simulink model "SoRo_Compliant_Demo_0906"  (R2023b)
settings: Solver=FixedStepAuto  StartTime=0.0  StopTime=inf  FixedStep=0.01  RelTol=1e-3
undefined symbols (not defined in the file): Down, Pull
libraries: simulink x50, speedgoatlib_IO691 x20, canmsglib x19, slpidlib x12, dspfdesign x6
(part 1 of 3)
settings Model: Creator=86188  LastModifiedBy=86188
settings SolverCC: ConcurrentTasks=on  PositivePriorityOrder=on
settings OptimizationCC: BlockReduction=off  OptimizeBlockIOStorage=off  BufferReuse=off
settings DebuggingCC: AlgebraicLoopMsg=none  TasksWithSamePriorityMsg=none
settings HardwareCC: ProdBitPerLong=64  ProdLongLongMode=on  ProdHWDeviceType=Intel->x86-64 (Linux 64)
settings RTWCC: Description=Simulink Real-Time  SystemTargetFile=slrealtime.tlc  TemplateMakefile=slrealtime_default_tmf  Toolchain=Simulink Real-Time Toolchain  BuildConfiguration=Faster Runs  CodeExecutionProfiling=on  TargetLang=C++

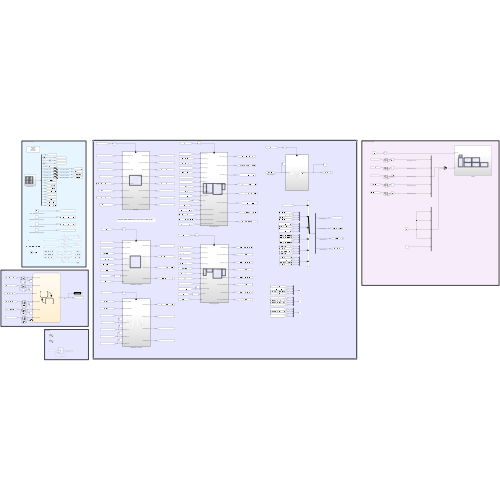
[thumbnail: Simulink's stored preview of the top-level diagram]
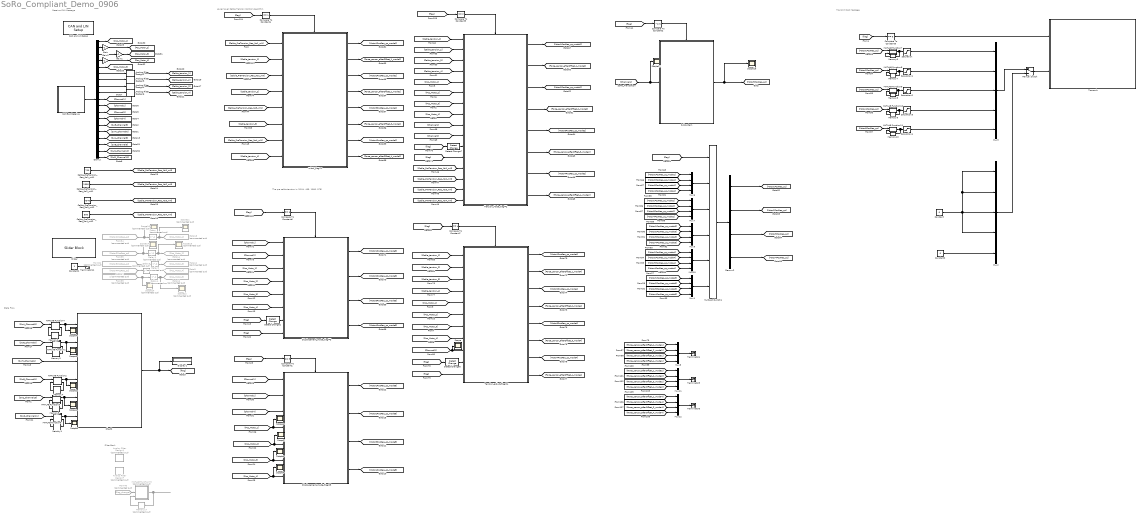
== system SoRo_Compliant_Demo_0906 ==
  note: Filter Bank
  note: Stata Flow
  note: Transmit CAN Message
  note: Receive CAN Message
  note: Lower level Cable Tension Control Algorithm
  note: The pre cable tension is (1104, 455, 1080, 978)
  Analog Filter Design1 : dspfdesign/Analog Filter Design  Commented=on  method=Chebyshev I  filttype=Lowpass  N=3  Wlo=1.5  Whi=80  Rp=2  Rs=40
  Analog Filter Design{2..4,6} (4 alike) : dspfdesign/Analog Filter Design  method=Butterworth  filttype=Lowpass  N=2  Wlo=1  Whi=80  Rp=2  Rs=40
  Analog Filter Design5 : dspfdesign/Analog Filter Design  Commented=on  method=Butterworth  filttype=Lowpass  N=3  Wlo=20  Whi=80  Rp=2  Rs=40
  CAN Bus Receive : Subsystem
  "CAN and LIN Setup " : speedgoatlib_IO691/CAN and LIN Setup   moduleInitValues="[691    1    1   -1   -1]"  id=1  moduleType=IO691  pciSlot=-1  canChn1=CAN (HS)  canChn2=CAN (HS)  canChn3=Disabled  canChn4=Disabled  linChn1=Disabled  linChn2=Disabled  canInitStructArray=[]  canTermStructArray=[]  gpioChnx=Disabled  canChn1InitValues="[2   2   8   1  16   3  19   2   2   5   2   0]"  arbBdrChn1=500 kBaud  clockDividerChn1=Enable  arbManBdrChn1=[8,1,16,3]  fdBdrChn1=5.0 MBaud  fdManBdrChn1=[2,2,5,2]  termResistor1=off  canChn2InitValues="[2   2   8   1  16   3  19   2   2   5   2   0]"  arbBdrChn2=500 kBaud  clockDividerChn2=Enable  arbManBdrChn2=[8,1,16,3]  fdBdrChn2=5.0 MBaud  fdManBdrChn2=[2,2,5,2]  termResistor2=off  canChn3InitValues="[1   0   2   8  31   8  19   2   2   5   2   0]"  arbBdrChn3=1.0 MBaud  clockDividerChn3=Enable  arbManBdrChn3=[2,8,31,8]  fdBdrChn3=5.0 MBaud  fdManBdrChn3=[2,2,5,2]  termResistor3=off  canChn4InitValues="[1   0   2   8  31   8  19   2   2   5   2   0]"  arbBdrChn4=1.0 MBaud  clockDividerChn4=Enable  arbManBdrChn4=[2,8,31,8]  fdBdrChn4=5.0 MBaud  fdManBdrChn4=[2,2,5,2]  termResistor4=off  linChn1InitValues="[0  9600]"  linBtrChn1=9600  linChn2InitValues="[0  9600]"  linBtrChn2=9600  doInitTermStruct="[0  5  0  0  0]"  parDoChannels=[1 2]  parDoVoltage=5  parDoInitValues=0  parDoReset=1  parNumOfDoS=0  parDiChannels=[3 4]  parDiVoltage=5  parDiPull=Pull-Down
      settings: SourceProductName=Simulink Real-Time: Speedgoat I/O Blockset
  Cable_PreTension_Req_No1_mN1 : Constant  Value=700
  Cable_PreTension_Req_No2_mN1 : Constant  Value=1300
  Cable_PreTension_Req_No3_mN2 : Constant  Value=7340
  Cable_PreTension_Req_No4_mN2 : Constant  Value=500
  Chart2 : Stateflow chart  TreatAsAtomicUnit=on
  Compare To Constant1 : simulink/Logic and Bit Operations/Compare To Constant  relop===  const=5  OutDataTypeStr=boolean
  Compare To Constant2 : simulink/Logic and Bit Operations/Compare To Constant  relop=~=  const=5  OutDataTypeStr=boolean
  Compare To Constant3 : simulink/Logic and Bit Operations/Compare To Constant  relop===  const=6  OutDataTypeStr=boolean
  Compare To Constant4 : simulink/Logic and Bit Operations/Compare To Constant  relop===  const=1  OutDataTypeStr=boolean
  Compare To Constant5 : simulink/Logic and Bit Operations/Compare To Constant  relop===  const=2  OutDataTypeStr=boolean
  Compare To Constant6 : simulink/Logic and Bit Operations/Compare To Constant  relop===  const=3  OutDataTypeStr=boolean
  Compare To Constant7 : simulink/Logic and Bit Operations/Compare To Constant  relop===  const=4  OutDataTypeStr=boolean
  Constant : Constant  Value=0
  Constant1 : Constant
  Constant2 : Constant  Value=0
  Delay{,1..4} (5 alike) : Delay  Commented=on
  Demux : Demux  Outputs=19
  Demux2 : Demux
  Detect Change1 : simulink/Logic and Bit Operations/Detect Change  vinit=0  OutDataTypeStr=boolean
  Detect Change6 : simulink/Logic and Bit Operations/Detect Change  vinit=0  OutDataTypeStr=boolean
  Detect Change7 : simulink/Logic and Bit Operations/Detect Change  vinit=0  OutDataTypeStr=boolean
  Displacement_mode_flag=3 : Subsystem
  Displacement_mode_flag=5 : Subsystem
  Display1 : Display
  From34 : From  Commented=on  GotoTag=Motor1PosReq_qc
  From35 : From  Commented=on  GotoTag=Motor2PosReq_qc
  From36 : From  Commented=on  GotoTag=Motor3PosReq_qc
  From37 : From  Commented=on  GotoTag=Motor4PosReq_qc
  From39 : From  Commented=on  GotoTag=Motor5PosReq_qc
  From40 : From  Commented=on  GotoTag=flag_change
  Gain : Gain  Gain=-1
  Gain1 : Gain  Gain=-1
  Gain2 : Gain  Gain=-1
  Goto12 : Goto  Commented=on  GotoTag=Pos_Motor_3
  Goto14 : Goto  Commented=on  GotoTag=Pos_Motor_2
  Goto16 : Goto  Commented=on  GotoTag=Pos_Motor_5
  Goto18 : Goto  Commented=on  GotoTag=Pos_Motor_1
  Goto9 : Goto  Commented=on  GotoTag=Pos_Motor_4
  Initial_flag=1 : Subsystem
  MATLAB Function1 : MATLAB Function  TreatAsAtomicUnit=on
  MATLAB Function10 : MATLAB Function  TreatAsAtomicUnit=on
  MATLAB Function11 : MATLAB Function  TreatAsAtomicUnit=on
  MATLAB Function13 : MATLAB Function  Commented=on  TreatAsAtomicUnit=on
  MATLAB Function2 : MATLAB Function  TreatAsAtomicUnit=on
  MATLAB Function3 : MATLAB Function  TreatAsAtomicUnit=on
  MATLAB Function4 : MATLAB Function  TreatAsAtomicUnit=on
  MATLAB Function6 : MATLAB Function  TreatAsAtomicUnit=on
  MATLAB Function7 : MATLAB Function  TreatAsAtomicUnit=on
  MATLAB Function8 : MATLAB Function  TreatAsAtomicUnit=on
  MATLAB Function9 : MATLAB Function  TreatAsAtomicUnit=on
  Manual Switch : ManualSwitch
  Memory{1..10} (10 alike) : Memory
  Memory17 : Memory  Commented=on
  Multiport Switch1 : MultiPortSwitch  Inputs=5  SaturateOnIntegerOverflow=off  InputSameDT=off
  Mux{1,6..12} (8 alike) : Mux
  Mux2 : Mux  Inputs=5
  Mux3 : Mux  Inputs=5
  Saturation{,1..3} (4 alike) : Saturate  UpperLimit=8000  LowerLimit=-8000
  Saturation4 : Saturate  UpperLimit=80000  LowerLimit=-80000
  Scope{,1..9,16..17} (12 alike) : Scope
  Scope{10..15} (6 alike) : Scope  Commented=on
  Slider : SliderBlock
  Subsystem : Subsystem
  Tension_Mode_flag=2 : Subsystem
  Tension_adjust_flag=4 : Subsystem
  Terminator{4..6,11} (4 alike) : Terminator
  Transmit : Subsystem
  wires:
  Mux8/1 -> Terminator4/1
  Tension_adjust_flag=4/5(Motor3PosReq_qc) -> [Motor3PosReq_qc_mode4]
  [flag] -> Detect Change6/1
  Demux/4 -> Gain2/1
  Tension_adjust_flag=4/1(Motor1PosReq_qc) -> [Motor1PosReq_qc_mode4]
  Tension_Mode_flag=2/8(Force_sensor_afterOffset_4) -> [Force_sensor_afterOffset_4_mode2]
  Multiport Switch1/1 -> Demux2/1
  [Motor1PosReq_qc_mode2] -> Mux7/1
  Manual Switch/1 -> Transmit/2(Input)
  [Motor2PosReq_qc_mode3] -> Mux9/2
  Tension_Mode_flag=2/1(Motor1_pos_req_qc) -> [Motor1PosReq_qc_mode2]
  [flag] -> Compare To Constant5/1
  [Motor1PosReq_qc_mode4] -> Mux10/1
  Tension_adjust_flag=4/4(Force_sensor_afterOffset_2) -> [Force_sensor_afterOffset_2_mode4]
  [Motor3PosReq_qc_mode2] -> Mux7/3
  Detect Change6/1 -> Tension_adjust_flag=4/10(flag_change)
  [Cable_tension_4] -> Tension_adjust_flag=4/4(Force_sensor_4_g)
  Tension_adjust_flag=4/3(Motor2_pos_req_qc) -> [Motor2PosReq_qc_mode4]
  [Motor2PosReq_qc_mode1] -> Mux6/2
  [Motor4PosReq_qc_mode1] -> Mux6/4
  Initial_flag=1/3(Motor2_pos_req_qc) -> [Motor2PosReq_qc_mode1]
  Mux9/1 -> Multiport Switch1/4
  Initial_flag=1/6(Force_sensor_afterOffset_3) -> [Force_sensor_afterOffset_3_mode1]
  Tension_adjust_flag=4/8(Force_sensor_afterOffset_4) -> [Force_sensor_afterOffset_4_mode4]
  [Force_sensor_afterOffset_1_mode4] -> Mux12/1
  [Force_sensor_afterOffset_1_mode1] -> Mux8/1
  [Channel3] -> Tension_adjust_flag=4/9(SoRo_Stifness_Adjust), Scope/1
  [Cable_PreTension_Req_No2_mN] -> Initial_flag=1/3(CableTension_Req_No2_mN)
  [Force_sensor_afterOffset_4_mode2] -> Mux11/4
  Initial_flag=1/5(Motor3PosReq_qc) -> [Motor3PosReq_qc_mode1]
  [Motor4PosReq_qc_mode3] -> Mux9/4
  [flag] -> Detect Change7/1
  Tension_Mode_flag=2/5(Motor3_pos_req_qc) -> [Motor3PosReq_qc_mode2]
  Compare To Constant5/1 -> Tension_Mode_flag=2/Enable
  [Force_sensor_afterOffset_2_mode2] -> Mux11/2
  [Force_sensor_afterOffset_3_mode1] -> Mux8/3
  [Motor1PosReq_qc_mode3] -> Mux9/1
  [Motor3PosReq_qc_mode3] -> Mux9/3
  [Motor2PosReq_qc_mode4] -> Mux10/2
  Tension_adjust_flag=4/7(Motor4PosReq_qc) -> [Motor4PosReq_qc_mode4]
  Tension_adjust_flag=4/6(Force_sensor_afterOffset_3) -> [Force_sensor_afterOffset_3_mode4]
  [Force_sensor_afterOffset_3_mode4] -> Mux12/3
  [flag] -> Compare To Constant4/1
  [Cable_tension_3] -> Tension_adjust_flag=4/3(Force_sensor_3_g)
  [Force_sensor_afterOffset_1_mode2] -> Mux11/1
  Mux12/1 -> Terminator6/1
  [Force_sensor_afterOffset_2_mode4] -> Mux12/2
  [Force_sensor_afterOffset_4_mode1] -> Mux8/4
  [Force_sensor_afterOffset_4_mode4] -> Mux12/4
  Displacement_mode_flag=3/3(Motor3PosReq_qc) -> [Motor3PosReq_qc_mode3]
  [Motor3PosReq_qc_mode4] -> Mux10/3
  Compare To Constant7/1 -> Tension_adjust_flag=4/Enable
  [flag] -> Tension_adjust_flag=4/11(flag)
  Mux11/1 -> Terminator5/1
  Detect Change7/1 -> Tension_Mode_flag=2/11(flag_change)
  [Cable_tension_1] -> Tension_adjust_flag=4/1(Force_sensor_1_g)
  Mux10/1 -> Multiport Switch1/5
  Displacement_mode_flag=3/2(Motor2_pos_req_qc) -> [Motor2PosReq_qc_mode3]
  Displacement_mode_flag=3/4(Motor4PosReq_qc) -> [Motor4PosReq_qc_mode3]
  [Motor3PosReq_qc] -> MATLAB Function9/1(u)
  Demux/3 -> Gain1/1
  Initial_flag=1/8(Force_sensor_afterOffset_4) -> [Force_sensor_afterOffset_4_mode1]
  [Cable_tension_2] -> Tension_adjust_flag=4/2(Force_sensor_2_g)
  [Channel2] -> Tension_Mode_flag=2/10(SoRo_Tip_Up/Down)
  Demux/7 -> Analog Filter Design3/1  "force_sensor_2_org"
  [flag] -> Compare To Constant3/1
  [Motor1PosReq_qc_mode1] -> Mux6/1
  [Cable_tension_3] -> Tension_Mode_flag=2/3(Force_sensor_3_g)
  [Channel2] -> Displacement_mode_flag=3/2(SoRo_Tip_Up/Down)
  Tension_Mode_flag=2/4(Force_sensor_afterOffset_2) -> [Force_sensor_afterOffset_2_mode2]
  Mux7/1 -> Multiport Switch1/3
  Tension_Mode_flag=2/2(Force_sensor_afterOffset_1) -> [Force_sensor_afterOffset_1_mode2]
  Tension_Mode_flag=2/3(Motor2_pos_req_qc) -> [Motor2PosReq_qc_mode2]
  [Motor4PosReq_qc_mode4] -> Mux10/4
  Displacement_mode_flag=3/1(Motor1PosReq_qc) -> [Motor1PosReq_qc_mode3]
  Initial_flag=1/7(Motor4PosReq_qc) -> [Motor4PosReq_qc_mode1]
  Tension_Mode_flag=2/7(Motor4_pos_req_qc) -> [Motor4PosReq_qc_mode2]
  [Force_sensor_afterOffset_2_mode1] -> Mux8/2
  [flag] -> Tension_Mode_flag=2/12(flag)
  [Force_sensor_afterOffset_3_mode2] -> Mux11/3
  [Cable_tension_2] -> Tension_Mode_flag=2/2(Force_sensor_2_g)
  [Cable_tension_4] -> Initial_flag=1/8(Force_sensor_4_g)
  [Channel1] -> Tension_Mode_flag=2/9(SoRo_Tip_Left/Right)
  Tension_adjust_flag=4/2(Force_sensor_afterOffset_1) -> [Force_sensor_afterOffset_1_mode4]
  Compare To Constant4/1 -> Initial_flag=1/Enable
  Tension_Mode_flag=2/6(Force_sensor_afterOffset_3) -> [Force_sensor_afterOffset_3_mode2]
  [flag] -> Compare To Constant6/1
  Mux6/1 -> Multiport Switch1/2
  [flag] -> Compare To Constant7/1
  [Cable_tension_3] -> Initial_flag=1/6(Force_sensor_3_g)
  [Motor3PosReq_qc_mode1] -> Mux6/3
  Demux/17 -> [SwB_Channel9]
  Mux2/1 -> Manual Switch/2
  Demux/1 -> [Pos_Motor_1]
  Demux/11 -> [Channel2]
  [Cable_tension_1] -> Tension_Mode_flag=2/1(Force_sensor_1_g)
  [Motor4PosReq_qc_mode2] -> Mux7/4
  [Cable_tension_4] -> Tension_Mode_flag=2/4(Force_sensor_4_g)
  [Cable_PreTension_Req_No3_mN] -> Initial_flag=1/5(CableTension_Req_No3_mN)
  Demux/16 -> [SwA_Channel8]
  [Motor2PosReq_qc_mode2] -> Mux7/2
  Compare To Constant6/1 -> Displacement_mode_flag=3/Enable
  [Cable_PreTension_Req_No1_mN] -> Initial_flag=1/1(CableTension_Req_No1_mN)
  Demux/9 -> Analog Filter Design6/1  "force_sensor_4_org"
  [Cable_tension_2] -> Initial_flag=1/4(Force_sensor_2_g)
  Demux/18 -> [SwC_Channel10]
  [Cable_tension_1] -> Initial_flag=1/2(Force_sensor_1_g)
  Demux/6 -> Analog Filter Design2/1  "force_sensor_1_org"
  Demux/13 -> [Channel4]
  Demux/15 -> [SwH_Channel6]
  Initial_flag=1/1(Motor1PosReq_qc) -> [Motor1PosReq_qc_mode1]
  [Channel1] -> Displacement_mode_flag=3/1(SoRo_Tip_Left/Right)
  Initial_flag=1/4(Force_sensor_afterOffset_2) -> [Force_sensor_afterOffset_2_mode1]
  Demux/8 -> Analog Filter Design4/1  "force_sensor_3_org"
  [Cable_PreTension_Req_No4_mN] -> Initial_flag=1/7(CableTension_Req_No4_mN)
  Demux/12 -> [Channel3]
  Initial_flag=1/2(Force_sensor_afterOffset_1) -> [Force_sensor_afterOffset_1_mode1]
  Demux/14 -> [SwE_Channel5]
  Demux/2 -> Gain/1
  CAN Bus Receive/1(Outport) -> Demux/1
  Demux/5 -> [Pos_Motor_5]
  Demux/10 -> [Channel1]
  [flag] -> Multiport Switch1/1
  MATLAB Function3/1(y) -> Chart2/5(Switch_C_Change), Scope1/1
  Memory5/1 -> MATLAB Function3/2(u_last)
  MATLAB Function4/1(y) -> Scope4/1, Chart2/1(Switch_A_Change)
  MATLAB Function3/2(u_out) -> Memory5/1
  MATLAB Function1/2(u_out) -> Memory3/1
  [SwC_Channel10] -> MATLAB Function3/1(u)
  MATLAB Function4/2(u_out) -> Memory2/1
  MATLAB Function2/2(u_out) -> Memory4/1
  Chart2/1(flag) -> Display1/1, [flag]  "flag"
  [SwH_Channel6] -> Chart2/3(Switch_H)
  MATLAB Function1/1(y) -> Scope3/1, Chart2/2(Switch_E_Change)
  Memory4/1 -> MATLAB Function2/2(u_last)
  [SwB_Channel9] -> MATLAB Function2/1(u)
  [SwA_Channel8] -> MATLAB Function4/1(u)
  Memory2/1 -> MATLAB Function4/2(u_last)
  Memory3/1 -> MATLAB Function1/2(u_last)
  [SwE_Channel5] -> MATLAB Function1/1(u)
  MATLAB Function2/1(y) -> Scope2/1, Chart2/4(Switch_B_Change)
  Compare To Constant3/1 -> Transmit/1(End Test)
  [Pos_Motor_2] -> Tension_Mode_flag=2/6(Pos_Motor_2_qc)
  [Pos_Motor_3] -> Tension_Mode_flag=2/7(Pos_Motor_3_qc)
  [Pos_Motor_4] -> Tension_Mode_flag=2/8(Pos_Motor_4_qc)
  [Pos_Motor_1] -> Tension_Mode_flag=2/5(Pos_Motor_1_qc)
  [Pos_Motor_3] -> Tension_adjust_flag=4/7(Pos_Motor_3_qc)
  [Pos_Motor_2] -> Tension_adjust_flag=4/6(Pos_Motor_2_qc)
  [Pos_Motor_4] -> Tension_adjust_flag=4/8(Pos_Motor_4_qc)
  [Pos_Motor_1] -> Tension_adjust_flag=4/5(Pos_Motor_1_qc)
  [Pos_Motor_2] -> Displacement_mode_flag=3/4(Pos_Motor_2_qc)
  [Pos_Motor_1] -> Displacement_mode_flag=3/3(Pos_Motor_1_qc)
  [Pos_Motor_3] -> Displacement_mode_flag=3/5(Pos_Motor_3_qc)
  [Pos_Motor_4] -> Displacement_mode_flag=3/6(Pos_Motor_4_qc)
  [flag] -> Detect Change1/1
  [flag] -> Displacement_mode_flag=3/8(flag)
  Detect Change1/1 -> Displacement_mode_flag=3/7(flag_change)
  Constant1/1 -> Terminator11/1
  MATLAB Function6/2(u_out) -> Memory1/1
  MATLAB Function6/1(y) -> Chart2/6(Switch_D_Change), Scope5/1
  [SwD_Channel11] -> MATLAB Function6/1(u)
  Memory1/1 -> MATLAB Function6/2(u_last)
  Demux/19 -> [SwD_Channel11]
  [Pos_Motor_1] -> Scope6/1, Displacement_mode_flag=5/4(Pos_Motor_1_qc)
  [Pos_Motor_4] -> Scope9/1, Displacement_mode_flag=5/7(Pos_Motor_4_qc)
  [flag] -> Compare To Constant1/1
  [Pos_Motor_3] -> Scope8/1, Displacement_mode_flag=5/6(Pos_Motor_3_qc)
  [Pos_Motor_2] -> Scope7/1, Displacement_mode_flag=5/5(Pos_Motor_2_qc)
  [Channel2] -> Displacement_mode_flag=5/2(UpMotor3_DownMotor2)
  [Channel1] -> Displacement_mode_flag=5/1(LeftMotor4_RightMotor1)
  Compare To Constant1/1 -> Displacement_mode_flag=5/Enable
  Displacement_mode_flag=5/1(Motor1PosReq_qc) -> [Motor1PosReq_qc_mode5]
  Displacement_mode_flag=5/3(Motor3PosReq_qc) -> [Motor3PosReq_qc_mode5]
  Displacement_mode_flag=5/4(Motor4PosReq_qc) -> [Motor4PosReq_qc_mode5]
  Displacement_mode_flag=5/2(Motor2_pos_req_qc) -> [Motor2PosReq_qc_mode5]
  [Channel4] -> Displacement_mode_flag=5/3(Pos_IncreaseDecrease)
  [Motor4PosReq_qc_mode5] -> Mux1/4
  [Motor3PosReq_qc_mode5] -> Mux1/3
  Mux1/1 -> Multiport Switch1/6
  [Motor2PosReq_qc_mode5] -> Mux1/2
  [Motor1PosReq_qc_mode5] -> Mux1/1
  Saturation4/1 -> Mux3/5  "Motor5PosReq_qc_final"
  Mux3/1 -> Manual Switch/1
  Saturation3/1 -> Mux3/4  "Motor4PosReq_qc_final"
  Saturation/1 -> Mux3/1  "Motor1PosReq_qc_final"
  Saturation1/1 -> Mux3/2  "Motor2PosReq_qc_final"
  Saturation2/1 -> Mux3/3  "Motor3PosReq_qc_final"
  [Motor1PosReq_qc] -> MATLAB Function7/1(u)
  MATLAB Function7/1(y) -> Memory6/1, Saturation/1
  Memory6/1 -> MATLAB Function7/2(u_last)
  MATLAB Function9/1(y) -> Memory8/1, Saturation2/1
  MATLAB Function8/1(y) -> Memory7/1, Saturation1/1
  [Motor2PosReq_qc] -> MATLAB Function8/1(u)
  Memory7/1 -> MATLAB Function8/2(u_last)
  Memory8/1 -> MATLAB Function9/2(u_last)
  MATLAB Function10/1(y) -> Memory9/1, Saturation3/1
  [Motor4PosReq_qc] -> MATLAB Function10/1(u)
  Memory9/1 -> MATLAB Function10/2(u_last)
  MATLAB Function11/1(y) -> Memory10/1, Saturation4/1
  Memory10/1 -> MATLAB Function11/2(u_last)
  From39/1 -> Delay4/1, Scope13/1
  From35/1 -> Delay1/1, Scope14/1
  From36/1 -> Delay2/1
  From37/1 -> Delay3/1
  Delay/1 -> Scope11/1, Goto18/1
  Delay1/1 -> Goto14/1, Scope15/1
  Delay2/1 -> Goto12/1
  Delay3/1 -> Goto9/1
  Delay4/1 -> Scope12/1, Goto16/1
  From40/1 -> MATLAB Function13/2(change)
  Memory17/1 -> MATLAB Function13/3(u_last)
  MATLAB Function13/1(y) -> Memory17/1  "Motor2PosReq_qc"
  Demux2/1 -> [Motor1PosReq_qc]  "Motor1PosReq_qc"
  Demux2/2 -> [Motor2PosReq_qc]  "Motor2PosReq_qc"
  Demux2/3 -> [Motor3PosReq_qc]  "Motor3PosReq_qc"
  Demux2/4 -> [Motor4PosReq_qc]  "Motor4PosReq_qc"
  From34/1 -> Scope10/1, Delay/1
  [Motor5PosReq_qc] -> MATLAB Function11/1(u)
  [Channel4] -> Scope17/1, Subsystem/1(Channel4)
  [flag] -> Compare To Constant2/1
  Compare To Constant2/1 -> Subsystem/Enable
  Subsystem/1(Motor5PosReq_qc) -> Scope16/1, [Motor5PosReq_qc]
  Analog Filter Design2/1 -> [Cable_tension_1]  "force_sensor_1_filtered"
  Analog Filter Design3/1 -> [Cable_tension_2]  "force_sensor_2_filtered"
  Analog Filter Design4/1 -> [Cable_tension_3]  "force_sensor_3_filtered"
  Analog Filter Design6/1 -> [Cable_tension_4]  "force_sensor_4_filtered"
  Constant/1 -> Mux2/4, Mux2/1, Mux2/2, Mux2/3
  Constant2/1 -> Mux2/5
  Gain/1 -> [Pos_Motor_2]
  Gain1/1 -> [Pos_Motor_3]
  Gain2/1 -> [Pos_Motor_4]
  Cable_PreTension_Req_No1_mN1/1 -> [Cable_PreTension_Req_No1_mN]
  Cable_PreTension_Req_No2_mN1/1 -> [Cable_PreTension_Req_No2_mN]
  Cable_PreTension_Req_No3_mN2/1 -> [Cable_PreTension_Req_No3_mN]
  Cable_PreTension_Req_No4_mN2/1 -> [Cable_PreTension_Req_No4_mN]
  [Cable_PreTension_Req_No1_mN] -> Tension_Mode_flag=2/13(Cable_PreTension_Req_No1_mN)
  [Cable_PreTension_Req_No2_mN] -> Tension_Mode_flag=2/14(Cable_PreTension_Req_No2_mN)
  [Cable_PreTension_Req_No3_mN] -> Tension_Mode_flag=2/15(Cable_PreTension_Req_No3_mN)
  [Cable_PreTension_Req_No4_mN] -> Tension_Mode_flag=2/16(Cable_PreTension_Req_No4_mN)

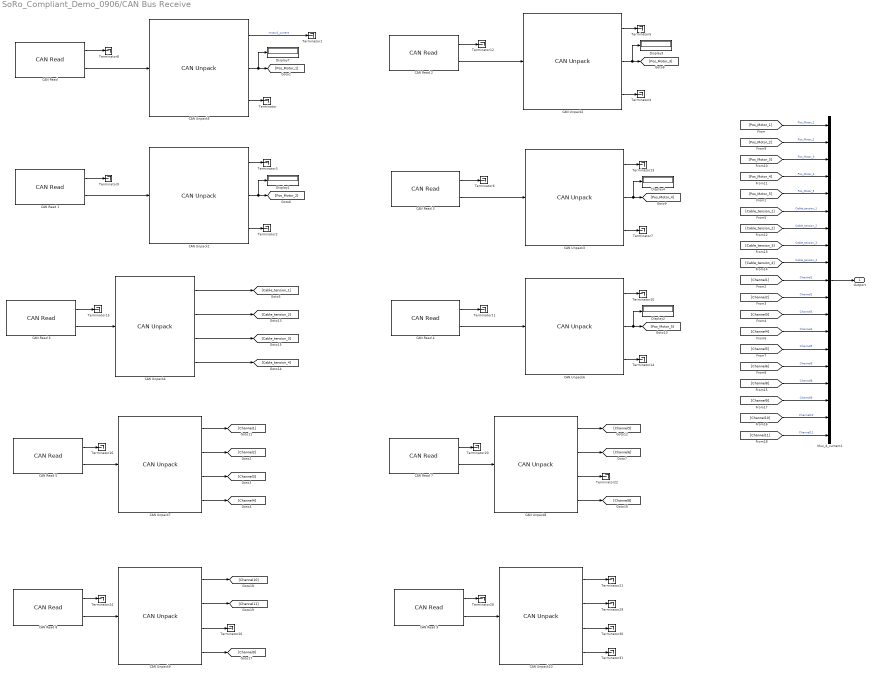
== system SoRo_Compliant_Demo_0906/CAN Bus Receive ==
  "CAN Read " : speedgoatlib_IO691/CAN Read   moduleType=IO691  id=1  channel=1  canType=CAN (HS)  messageType=CAN (HS)  useBusOut=off  HasMulRead=Specify by IDs  MsgIDlist=[27]  isEFF=off  LabelInHex=on  enableInput=off  initValues=[691 1 0.01 0 1 1 0 0 2 0 1 27]  ts=0.01
      settings: SourceProductName=Simulink Real-Time: Speedgoat I/O Blockset
  CAN Read 1 : speedgoatlib_IO691/CAN Read   moduleType=IO691  id=1  channel=1  canType=CAN (HS)  messageType=CAN (HS)  useBusOut=off  HasMulRead=Specify by IDs  MsgIDlist=[43]  isEFF=off  LabelInHex=on  enableInput=off  initValues=[691 1 0.01 0 1 1 0 0 2 0 1 43]  ts=0.01
      settings: SourceProductName=Simulink Real-Time: Speedgoat I/O Blockset
  CAN Read 2 : speedgoatlib_IO691/CAN Read   moduleType=IO691  id=1  channel=1  canType=CAN (HS)  messageType=CAN (HS)  useBusOut=off  HasMulRead=Specify by IDs  MsgIDlist=[59]  isEFF=off  LabelInHex=on  enableInput=off  initValues=[691 1 0.01 0 1 1 0 0 2 0 1 59]  ts=0.01
      settings: SourceProductName=Simulink Real-Time: Speedgoat I/O Blockset
  CAN Read 3 : speedgoatlib_IO691/CAN Read   moduleType=IO691  id=1  channel=1  canType=CAN (HS)  messageType=CAN (HS)  useBusOut=off  HasMulRead=Specify by IDs  MsgIDlist=[75]  isEFF=off  LabelInHex=on  enableInput=off  initValues=[691 1 0.01 0 1 1 0 0 2 0 1 75]  ts=0.01
      settings: SourceProductName=Simulink Real-Time: Speedgoat I/O Blockset
  CAN Read 4 : speedgoatlib_IO691/CAN Read   moduleType=IO691  id=1  channel=1  canType=CAN (HS)  messageType=CAN (HS)  useBusOut=off  HasMulRead=Specify by IDs  MsgIDlist=[91]  isEFF=off  LabelInHex=on  enableInput=off  initValues=[691 1 0.01 0 1 1 0 0 2 0 1 91]  ts=0.01
      settings: SourceProductName=Simulink Real-Time: Speedgoat I/O Blockset
  CAN Read 5 : speedgoatlib_IO691/CAN Read   moduleType=IO691  id=1  channel=1  canType=CAN (HS)  messageType=CAN (HS)  useBusOut=off  HasMulRead=Specify by IDs  MsgIDlist=[391]  isEFF=off  LabelInHex=on  enableInput=off  initValues=[691 1 0.01 0 1 1 0 0 2 0 1 391]  ts=0.01
      settings: SourceProductName=Simulink Real-Time: Speedgoat I/O Blockset
  CAN Read 6 : speedgoatlib_IO691/CAN Read   moduleType=IO691  id=1  channel=1  canType=CAN (HS)  messageType=CAN (HS)  useBusOut=off  HasMulRead=Specify by IDs  MsgIDlist=[529024]  isEFF=on  LabelInHex=on  enableInput=off  initValues=[691 1 0.01 0 1 1 0 0 2 1 1 529024]  ts=0.01
      settings: SourceProductName=Simulink Real-Time: Speedgoat I/O Blockset
  CAN Read 7 : speedgoatlib_IO691/CAN Read   moduleType=IO691  id=1  channel=1  canType=CAN (HS)  messageType=CAN (HS)  useBusOut=off  HasMulRead=Specify by IDs  MsgIDlist=[392]  isEFF=off  LabelInHex=on  enableInput=off  initValues=[691 1 0.01 0 1 1 0 0 2 0 1 392]  ts=0.01
      settings: SourceProductName=Simulink Real-Time: Speedgoat I/O Blockset
  CAN Read 8 : speedgoatlib_IO691/CAN Read   moduleType=IO691  id=1  channel=1  canType=CAN (HS)  messageType=CAN (HS)  useBusOut=off  HasMulRead=Specify by IDs  MsgIDlist=[393]  isEFF=off  LabelInHex=on  enableInput=off  initValues=[691 1 0.01 0 1 1 0 0 2 0 1 393]  ts=0.01
      settings: SourceProductName=Simulink Real-Time: Speedgoat I/O Blockset
  CAN Read 9 : speedgoatlib_IO691/CAN Read   moduleType=IO691  id=1  channel=1  canType=CAN (HS)  messageType=CAN (HS)  useBusOut=off  HasMulRead=Specify by IDs  MsgIDlist=[394]  isEFF=off  LabelInHex=on  enableInput=off  initValues=[691 1 0.01 0 1 1 0 0 2 0 1 394]  ts=0.01
      settings: SourceProductName=Simulink Real-Time: Speedgoat I/O Blockset
  CAN Unpack1 : canmsglib/CAN Unpack  CANdbFile=E:\OneDrive\OneDrive - The Chinese University of Hong Kong\文档\Research\SRIL\12nd\Experiment\Simulink\RoboModule0729.dbc  MsgList=Feedback_curvelpos_Dv2  MsgName=Feedback_curvelpos_Dv2  MsgIDType=Standard (11-bit identifier)  MsgIdentifier=43  MsgLength=8  SignalInfo={'real_current','8','16','BE','signed','Standard','0','1','0','-Inf','Inf';'real_position','56','32','BE','signed','Standard','0','1','0','-Inf','Inf';'real_velocity','24','16','BE','signed','Standard','0','1','0','-Inf','Inf'}  IDPort=off  TimestampPort=off  ErrorPort=off  RemotePort=off  LengthPort=off  StatusPort=off  ApplyMinMax=off
      settings: DataFormat=CANdb specified signals
  CAN Unpack10 : canmsglib/CAN Unpack  CANdbFile=E:\OneDrive\OneDrive - The Chinese University of Hong Kong\文档\Research\SRIL\12nd\Experiment\Simulink\RoboModule0729.dbc  MsgList=RadioLink_4  MsgName=RadioLink_4  MsgIDType=Standard (11-bit identifier)  MsgIdentifier=394  MsgLength=8  SignalInfo={'Channel13','8','16','BE','unsigned','Standard','0','1','0','-Inf','Inf';'Channel14','24','16','BE','unsigned','Standard','0','1','0','-Inf','Inf';'Channel15','40','16','BE','unsigned','Standard','0','1','0','-Inf','Inf';'Channel16','56','16','BE','unsigned','Standard','0','1','0','-Inf','Inf'}  IDPort=off  TimestampPort=off  ErrorPort=off  RemotePort=off  LengthPort=off  StatusPort=off  ApplyMinMax=off
      settings: DataFormat=CANdb specified signals
  CAN Unpack2 : canmsglib/CAN Unpack  CANdbFile=E:\OneDrive\OneDrive - The Chinese University of Hong Kong\文档\Research\SRIL\12nd\Experiment\Simulink\RoboModule0729.dbc  MsgList=Feedback_curvelpos_Dv3  MsgName=Feedback_curvelpos_Dv3  MsgIDType=Standard (11-bit identifier)  MsgIdentifier=59  MsgLength=8  SignalInfo={'real_current','8','16','BE','signed','Standard','0','1','0','-Inf','Inf';'real_position','56','32','BE','signed','Standard','0','1','0','-Inf','Inf';'real_velocity','24','16','BE','signed','Standard','0','1','0','-Inf','Inf'}  IDPort=off  TimestampPort=off  ErrorPort=off  RemotePort=off  LengthPort=off  StatusPort=off  ApplyMinMax=off
      settings: DataFormat=CANdb specified signals
  CAN Unpack3 : canmsglib/CAN Unpack  CANdbFile=E:\OneDrive\OneDrive - The Chinese University of Hong Kong\文档\Research\SRIL\12nd\Experiment\Simulink\RoboModule0729.dbc  MsgList=Feedback_curvelpos_Dr4  MsgName=Feedback_curvelpos_Dr4  MsgIDType=Standard (11-bit identifier)  MsgIdentifier=75  MsgLength=8  SignalInfo={'real_current','8','16','BE','signed','Standard','0','1','0','-Inf','Inf';'real_position','56','32','BE','signed','Standard','0','1','0','-Inf','Inf';'real_velocity','24','16','BE','signed','Standard','0','1','0','-Inf','Inf'}  IDPort=off  TimestampPort=off  ErrorPort=off  RemotePort=off  LengthPort=off  StatusPort=off  ApplyMinMax=off
      settings: DataFormat=CANdb specified signals
  CAN Unpack4 : canmsglib/CAN Unpack  CANdbFile=E:\OneDrive\OneDrive - The Chinese University of Hong Kong\文档\Research\SRIL\12nd\Experiment\Simulink\RoboModule0729.dbc  MsgList=Cable_tension  MsgName=Cable_tension  MsgIDType=Extended (29-bit identifier)  MsgIdentifier=529024  MsgLength=8  SignalInfo={'Force_sensor_1','8','16','BE','unsigned','Standard','0','1','0','-Inf','Inf';'Force_sensor_2','24','16','BE','unsigned','Standard','0','1','0','-Inf','Inf';'Force_sensor_3','40','16','BE','unsigned','Standard','0','1','0','-Inf','Inf';'Force_sensor_4','56','16','BE','unsigned','Standard','0','1','0','-Inf','Inf'}  IDPort=off  TimestampPort=off  ErrorPort=off  RemotePort=off  LengthPort=off  StatusPort=off  ApplyMinMax=off
      settings: DataFormat=CANdb specified signals
  CAN Unpack5 : canmsglib/CAN Unpack  CANdbFile=E:\OneDrive\OneDrive - The Chinese University of Hong Kong\文档\Research\SRIL\12nd\Experiment\Simulink\RoboModule0729.dbc  MsgList=Feedback_curvelpos_Dv1  MsgName=Feedback_curvelpos_Dv1  MsgIDType=Standard (11-bit identifier)  MsgIdentifier=27  MsgLength=8  SignalInfo={'real_current','8','16','BE','signed','Standard','0','1','0','-Inf','Inf';'real_position','56','32','BE','signed','Standard','0','1','0','-Inf','Inf';'real_velocity','24','16','BE','signed','Standard','0','1','0','-Inf','Inf'}  IDPort=off  TimestampPort=off  ErrorPort=off  RemotePort=off  LengthPort=off  StatusPort=off  ApplyMinMax=off
      settings: DataFormat=CANdb specified signals
  CAN Unpack6 : canmsglib/CAN Unpack  CANdbFile=E:\OneDrive\OneDrive - The Chinese University of Hong Kong\文档\Research\SRIL\12nd\Experiment\Simulink\RoboModule0729.dbc  MsgList=Feedback_curvelpos_Dr5  MsgName=Feedback_curvelpos_Dr5  MsgIDType=Standard (11-bit identifier)  MsgIdentifier=91  MsgLength=8  SignalInfo={'real_current','8','16','BE','signed','Standard','0','1','0','-Inf','Inf';'real_position','56','32','BE','signed','Standard','0','1','0','-Inf','Inf';'real_velocity','24','16','BE','signed','Standard','0','1','0','-Inf','Inf'}  IDPort=off  TimestampPort=off  ErrorPort=off  RemotePort=off  LengthPort=off  StatusPort=off  ApplyMinMax=off
      settings: DataFormat=CANdb specified signals
  CAN Unpack7 : canmsglib/CAN Unpack  CANdbFile=E:\OneDrive\OneDrive - The Chinese University of Hong Kong\文档\Research\SRIL\12nd\Experiment\Simulink\RoboModule0729.dbc  MsgList=RadioLink_1  MsgName=RadioLink_1  MsgIDType=Standard (11-bit identifier)  MsgIdentifier=391  MsgLength=8  SignalInfo={'Channel1','8','16','BE','unsigned','Standard','0','1','0','-Inf','Inf';'Channel2','24','16','BE','unsigned','Standard','0','1','0','-Inf','Inf';'Channel3','40','16','BE','unsigned','Standard','0','1','0','-Inf','Inf';'Channel4','56','16','BE','unsigned','Standard','0','1','0','-Inf','Inf'}  IDPort=off  TimestampPort=off  ErrorPort=off  RemotePort=off  LengthPort=off  StatusPort=off  ApplyMinMax=off
      settings: DataFormat=CANdb specified signals
  CAN Unpack8 : canmsglib/CAN Unpack  CANdbFile=E:\OneDrive\OneDrive - The Chinese University of Hong Kong\文档\Research\SRIL\12nd\Experiment\Simulink\RoboModule0729.dbc  MsgList=RadioLink_2  MsgName=RadioLink_2  MsgIDType=Standard (11-bit identifier)  MsgIdentifier=392  MsgLength=8  SignalInfo={'Channel5','8','16','BE','unsigned','Standard','0','1','0','-Inf','Inf';'Channel6','24','16','BE','unsigned','Standard','0','1','0','-Inf','Inf';'Channel7','40','16','BE','unsigned','Standard','0','1','0','-Inf','Inf';'Channel8','56','16','BE','unsigned','Standard','0','1','0','-Inf','Inf'}  IDPort=off  TimestampPort=off  ErrorPort=off  RemotePort=off  LengthPort=off  StatusPort=off  ApplyMinMax=off
      settings: DataFormat=CANdb specified signals
  CAN Unpack9 : canmsglib/CAN Unpack  CANdbFile=E:\Research\SRIL\12nd\Simulink\RoboModule0729.dbc  MsgList=RadioLink_3  MsgName=RadioLink_3  MsgIDType=Standard (11-bit identifier)  MsgIdentifier=393  MsgLength=8  SignalInfo={'Channel10','24','16','BE','unsigned','Standard','0','1','0','-Inf','Inf';'Channel11','40','16','BE','unsigned','Standard','0','1','0','-Inf','Inf';'Channel12','56','16','BE','unsigned','Standard','0','1','0','-Inf','Inf';'Channel9','8','16','BE','unsigned','Standard','0','1','0','-Inf','Inf'}  IDPort=off  TimestampPort=off  ErrorPort=off  RemotePort=off  LengthPort=off  StatusPort=off  ApplyMinMax=off
      settings: DataFormat=CANdb specified signals
  Display{1..4,7} (5 alike) : Display
      settings: Format=hex (Stored Integer)
  Mux_4_current1 : Mux  Inputs=19
  Terminator{,1..16,20..22,24,26,28..31} (26 alike) : Terminator
  Outport : Outport
  wires:
  CAN Unpack5/3 -> Terminator/1
  CAN Unpack4/1 -> [Cable_tension_1]
  CAN Unpack5/1 -> Terminator1/1  "motor1_current"
  "CAN Read "/2 -> CAN Unpack5/1
  CAN Unpack4/2 -> [Cable_tension_2]
  CAN Unpack5/2 -> Display7/1, [Pos_Motor_1]
  "CAN Read "/1 -> Terminator8/1
  CAN Read 1/2 -> CAN Unpack1/1
  CAN Read 1/1 -> Terminator9/1
  CAN Unpack1/2 -> Display1/1, [Pos_Motor_2]
  CAN Unpack1/3 -> Terminator2/1
  CAN Unpack1/1 -> Terminator3/1
  CAN Read 2/2 -> CAN Unpack2/1
  CAN Read 2/1 -> Terminator12/1
  CAN Unpack2/3 -> Terminator4/1
  CAN Unpack2/2 -> Display3/1, [Pos_Motor_3]
  CAN Unpack2/1 -> Terminator5/1
  CAN Read 3/2 -> CAN Unpack3/1
  CAN Unpack3/3 -> Terminator7/1
  CAN Read 3/1 -> Terminator6/1
  CAN Unpack3/1 -> Terminator13/1
  CAN Unpack3/2 -> Display4/1, [Pos_Motor_4]
  CAN Unpack6/2 -> Display2/1, [Pos_Motor_5]
  CAN Read 4/2 -> CAN Unpack6/1
  CAN Unpack6/1 -> Terminator10/1
  CAN Read 4/1 -> Terminator11/1
  CAN Unpack6/3 -> Terminator14/1
  CAN Read 6/1 -> Terminator15/1
  CAN Read 6/2 -> CAN Unpack4/1
  CAN Read 5/1 -> Terminator16/1
  CAN Read 5/2 -> CAN Unpack7/1
  CAN Unpack7/1 -> [Channel1]
  CAN Unpack7/2 -> [Channel2]
  CAN Unpack7/3 -> [Channel3]
  CAN Unpack7/4 -> [Channel4]
  CAN Unpack8/4 -> [Channel8]
  CAN Read 7/1 -> Terminator20/1
  CAN Unpack8/1 -> [Channel5]
  CAN Unpack8/2 -> [Channel6]
  CAN Read 7/2 -> CAN Unpack8/1
  CAN Unpack8/3 -> Terminator22/1
  CAN Unpack9/3 -> Terminator26/1
  CAN Unpack9/1 -> [Channel10]
  CAN Read 8/2 -> CAN Unpack9/1
  CAN Read 8/1 -> Terminator24/1
  CAN Unpack9/2 -> [Channel11]
  CAN Unpack9/4 -> [Channel9]
  CAN Unpack10/2 -> Terminator29/1
  CAN Read 9/1 -> Terminator28/1
  CAN Unpack10/4 -> Terminator31/1
  CAN Read 9/2 -> CAN Unpack10/1
  CAN Unpack10/3 -> Terminator30/1
  CAN Unpack10/1 -> Terminator21/1
  [Channel1] -> Mux_4_current1/10  "Channel1"
  [Channel2] -> Mux_4_current1/11  "Channel2"
  [Channel4] -> Mux_4_current1/13  "Channel4"
  [Channel3] -> Mux_4_current1/12  "Channel3"
  [Channel5] -> Mux_4_current1/14  "Channel5"
  [Channel6] -> Mux_4_current1/15  "Channel6"
  CAN Unpack4/4 -> [Cable_tension_4]
  CAN Unpack4/3 -> [Cable_tension_3]
  [Pos_Motor_1] -> Mux_4_current1/1  "Pos_Motor_1"
  Mux_4_current1/1 -> Outport/1
  [Pos_Motor_2] -> Mux_4_current1/2  "Pos_Motor_2"
  [Pos_Motor_3] -> Mux_4_current1/3  "Pos_Motor_3"
  [Pos_Motor_4] -> Mux_4_current1/4  "Pos_Motor_4"
  [Pos_Motor_5] -> Mux_4_current1/5  "Pos_Motor_5"
  [Cable_tension_1] -> Mux_4_current1/6  "Cable_tension_1"
  [Cable_tension_2] -> Mux_4_current1/7  "Cable_tension_2"
  [Cable_tension_3] -> Mux_4_current1/8  "Cable_tension_3"
  [Cable_tension_4] -> Mux_4_current1/9  "Cable_tension_4"
  [Channel8] -> Mux_4_current1/16  "Channel8"
  [Channel10] -> Mux_4_current1/18  "Channel10"
  [Channel9] -> Mux_4_current1/17  "Channel9"
  [Channel11] -> Mux_4_current1/19  "Channel11"

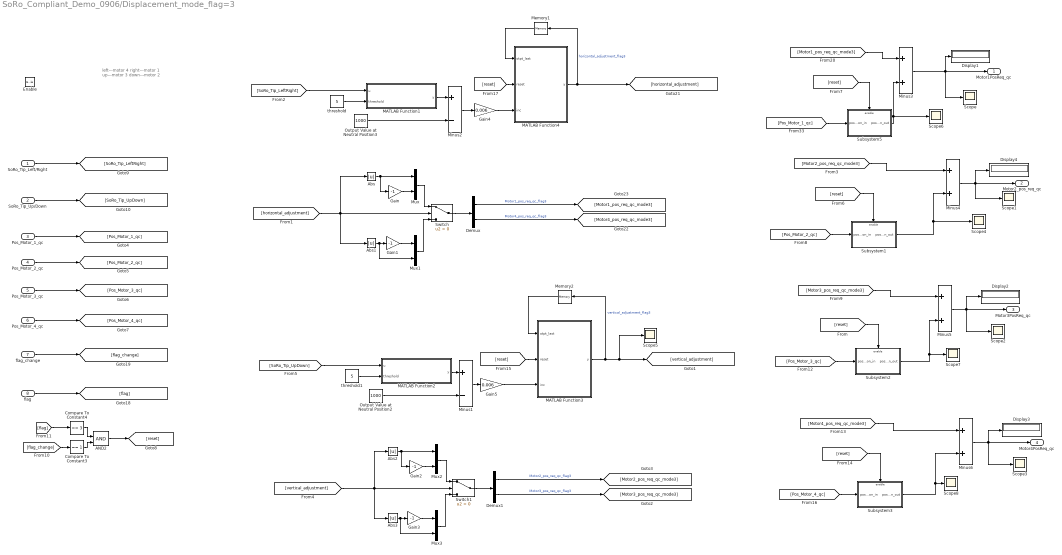
== system SoRo_Compliant_Demo_0906/Displacement_mode_flag=3 ==
  note: left---motor 4
      | right---motor 1
      | up---motor 3
      | down---motor 2
  SoRo_Tip_Left/Right : Inport
  SoRo_Tip_Up/Down : Inport  Port=2
  Pos_Motor_1_qc : Inport  Port=3
  Pos_Motor_2_qc : Inport  Port=4
  Pos_Motor_3_qc : Inport  Port=5
  Pos_Motor_4_qc : Inport  Port=6
  flag_change : Inport  Port=7
  flag : Inport  Port=8
  Enable : EnablePort  StatesWhenEnabling=reset
  AND2 : Logic  IconShape=distinctive  AllPortsSameDT=off  OutDataTypeStr=boolean
  Abs{,1..3} (4 alike) : Abs  SaturateOnIntegerOverflow=off
  Compare To Constant3 : simulink/Logic and Bit Operations/Compare To Constant  relop===  const=1  OutDataTypeStr=boolean
  Compare To Constant4 : simulink/Logic and Bit Operations/Compare To Constant  relop===  const=3  OutDataTypeStr=boolean
  Demux : Demux  Outputs=2
  Demux1 : Demux  Outputs=2
  Display{1..4} (4 alike) : Display
  Gain{,1..3} (4 alike) : Gain  Gain=-1
  Gain4 : Gain  Gain=0.006
  Gain5 : Gain  Gain=0.006
  MATLAB Function1 : MATLAB Function  TreatAsAtomicUnit=on
  MATLAB Function2 : MATLAB Function  TreatAsAtomicUnit=on
  MATLAB Function3 : MATLAB Function  TreatAsAtomicUnit=on
  MATLAB Function4 : MATLAB Function  TreatAsAtomicUnit=on
  Memory1 : Memory
  Memory2 : Memory
  Minus1 : Sum  Inputs=+-
  Minus2 : Sum  Inputs=+-
  Minus{3..6} (4 alike) : Sum
  Mux{,1..3} (4 alike) : Mux  Inputs=2
  Output Value at Neutral Position2 : Constant  Value=1000
  Output Value at Neutral Position3 : Constant  Value=1000
  Scope{,1..8} (9 alike) : Scope
  Subsystem1 : Subsystem
  Subsystem2 : Subsystem
  Subsystem3 : Subsystem
  Subsystem5 : Subsystem
  Switch : Switch  Criteria=u2 > Threshold  SaturateOnIntegerOverflow=off  InputSameDT=off
  Switch1 : Switch  Criteria=u2 > Threshold  SaturateOnIntegerOverflow=off  InputSameDT=off
  threshold : Constant  Value=5
  threshold1 : Constant  Value=5
  Motor1PosReq_qc : Outport
  Motor2_pos_req_qc : Outport  Port=2
  Motor3PosReq_qc : Outport  Port=3
  Motor4PosReq_qc : Outport  Port=4
  wires:
  SoRo_Tip_Left/Right/1 -> [SoRo_Tip_LeftRight]
  SoRo_Tip_Up/Down/1 -> [SoRo_Tip_UpDown]
  Minus2/1 -> Gain4/1
  Demux/1 -> [Motor1_pos_req_qc_mode3]  "Motor1_pos_req_qc_flag3"
  Demux/2 -> [Motor4_pos_req_qc_mode3]  "Motor4_pos_req_qc_flag3"
  Switch/1 -> Demux/1
  Gain/1 -> Mux/2
  Abs/1 -> Gain/1, Mux/1
  Mux/1 -> Switch/1
  Abs1/1 -> Mux1/2, Gain1/1
  [horizontal_adjustment] -> Abs1/1, Abs/1, Switch/2
  Mux1/1 -> Switch/3
  Demux1/2 -> [Motor3_pos_req_qc_mode3]  "Motor3_pos_req_qc_flag3"
  Switch1/1 -> Demux1/1
  Minus1/1 -> Gain5/1
  Output Value at Neutral Position2/1 -> Minus1/2
  Abs3/1 -> Mux3/2, Gain3/1
  [vertical_adjustment] -> Abs3/1, Abs2/1, Switch1/2
  Demux1/1 -> [Motor2_pos_req_qc_mode3]  "Motor2_pos_req_qc_flag3"
  Mux3/1 -> Switch1/3
  MATLAB Function3/1(y) -> Memory2/1, Scope5/1, [vertical_adjustment]  "vertical_adjustment_flag3"
  Abs2/1 -> Gain2/1, Mux2/1
  Gain2/1 -> Mux2/2
  [SoRo_Tip_LeftRight] -> MATLAB Function1/1(u)
  MATLAB Function1/1(y) -> Minus2/1
  threshold/1 -> MATLAB Function1/2(threshold)
  Output Value at Neutral Position3/1 -> Minus2/2
  Gain1/1 -> Mux1/1
  threshold1/1 -> MATLAB Function2/2(threshold)
  [SoRo_Tip_UpDown] -> MATLAB Function2/1(u)
  MATLAB Function2/1(y) -> Minus1/1
  Mux2/1 -> Switch1/1
  Gain3/1 -> Mux3/1
  Pos_Motor_4_qc/1 -> [Pos_Motor_4_qc]
  Pos_Motor_3_qc/1 -> [Pos_Motor_3_qc]
  Pos_Motor_2_qc/1 -> [Pos_Motor_2_qc]
  Pos_Motor_1_qc/1 -> [Pos_Motor_1_qc]
  flag/1 -> [flag]
  flag_change/1 -> [flag_change]
  [Pos_Motor_1_qc] -> Subsystem5/1(position_in)
  [reset] -> Subsystem5/Enable
  [Motor1_pos_req_qc_mode3] -> Minus3/1
  Minus3/1 -> Scope/1, Display1/1, Motor1PosReq_qc/1
  Subsystem5/1(position_out) -> Minus3/2, Scope6/1
  [Motor2_pos_req_qc_mode3] -> Minus4/1
  [reset] -> Subsystem1/Enable
  [Pos_Motor_2_qc] -> Subsystem1/1(position_in)
  Minus4/1 -> Scope1/1, Display4/1, Motor2_pos_req_qc/1
  Minus5/1 -> Scope2/1, Motor3PosReq_qc/1, Display2/1
  [reset] -> Subsystem2/Enable
  [Pos_Motor_3_qc] -> Subsystem2/1(position_in)
  [Motor3_pos_req_qc_mode3] -> Minus5/1
  Minus6/1 -> Scope3/1, Motor4PosReq_qc/1, Display3/1
  [reset] -> Subsystem3/Enable
  [Pos_Motor_4_qc] -> Subsystem3/1(position_in)
  [Motor4_pos_req_qc_mode3] -> Minus6/1
  MATLAB Function4/1(y) -> [horizontal_adjustment], Memory1/1  "horizontal_adjustment_flag3"
  Compare To Constant4/1 -> AND2/1
  Compare To Constant3/1 -> AND2/2
  [flag_change] -> Compare To Constant3/1
  [flag] -> Compare To Constant4/1
  AND2/1 -> [reset]
  [reset] -> MATLAB Function3/2(reset)
  Memory1/1 -> MATLAB Function4/1(otpt_last)
  [reset] -> MATLAB Function4/2(reset)
  Gain4/1 -> MATLAB Function4/3(inc)
  Subsystem2/1(position_out) -> Minus5/2, Scope7/1
  Subsystem3/1(position_out) -> Minus6/2, Scope8/1
  Subsystem1/1(position_out) -> Minus4/2, Scope4/1
  Gain5/1 -> MATLAB Function3/3(inc)
  Memory2/1 -> MATLAB Function3/1(otpt_last)

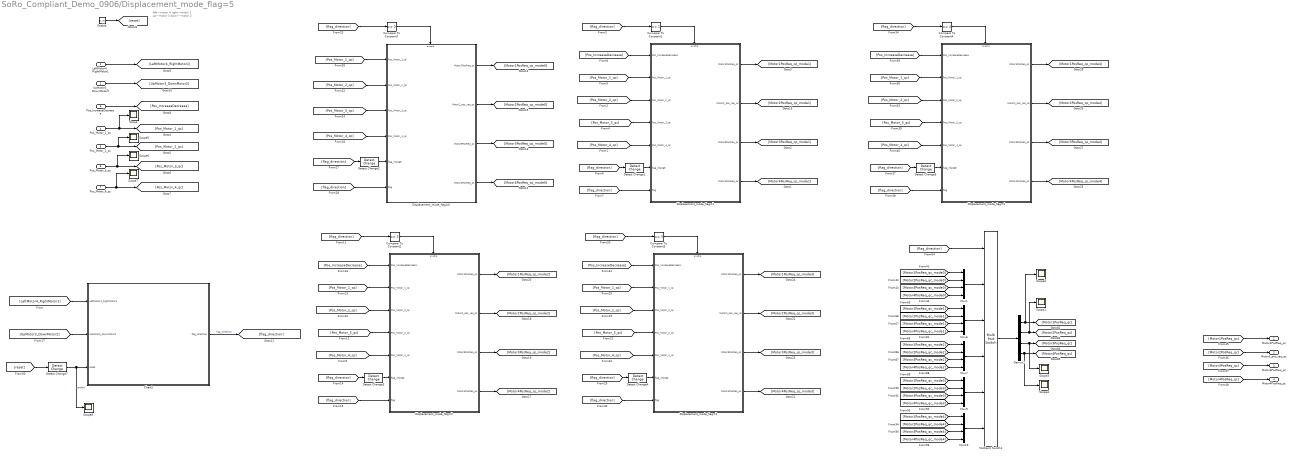
== system SoRo_Compliant_Demo_0906/Displacement_mode_flag=5 ==
  note: left---motor 4
      | right---motor 1
      | up---motor 3
      | down---motor 2
  LeftMotor4_RightMotor1 : Inport
  UpMotor3_DownMotor2 : Inport  Port=2
  Pos_IncreaseDecrease : Inport  Port=3
  Pos_Motor_1_qc : Inport  Port=4
  Pos_Motor_2_qc : Inport  Port=5
  Pos_Motor_3_qc : Inport  Port=6
  Pos_Motor_4_qc : Inport  Port=7
  Enable : EnablePort  StatesWhenEnabling=reset  ShowOutputPort=on
  Chart2 : Stateflow chart  TreatAsAtomicUnit=on
  Compare To Constant1 : simulink/Logic and Bit Operations/Compare To Constant  relop===  const=1  OutDataTypeStr=boolean
  Compare To Constant2 : simulink/Logic and Bit Operations/Compare To Constant  relop===  const=2  OutDataTypeStr=boolean
  Compare To Constant3 : simulink/Logic and Bit Operations/Compare To Constant  relop===  const=3  OutDataTypeStr=boolean
  Compare To Constant4 : simulink/Logic and Bit Operations/Compare To Constant  relop===  const=4  OutDataTypeStr=boolean
  Compare To Constant7 : simulink/Logic and Bit Operations/Compare To Constant  relop===  const=0  OutDataTypeStr=boolean
  Demux2 : Demux
  Detect Change{1..5,7} (6 alike) : simulink/Logic and Bit Operations/Detect Change  vinit=0  OutDataTypeStr=boolean
  Displacement_mode_flag=0 : Subsystem
  Displacement_mode_flag=1 : Subsystem
  Displacement_mode_flag=2 : Subsystem
  Displacement_mode_flag=3 : Subsystem
  Displacement_mode_flag=4 : Subsystem
  Multiport Switch1 : MultiPortSwitch  DataPortOrder=Zero-based contiguous  Inputs=5  zeroidx=on  SaturateOnIntegerOverflow=off  InputSameDT=off
  Mux{1,6..7,9..10} (5 alike) : Mux
  Scope{,1..8} (9 alike) : Scope
  Motor1PosReq_qc : Outport
  Motor2_pos_req_qc : Outport  Port=2
  Motor3PosReq_qc : Outport  Port=3
  Motor4PosReq_qc : Outport  Port=4
  wires:
  LeftMotor4_RightMotor1/1 -> [LeftMotor4_RightMotor1]
  UpMotor3_DownMotor2/1 -> [UpMotor3_DownMotor2]
  Pos_Motor_4_qc/1 -> Scope7/1, [Pos_Motor_4_qc]
  Pos_Motor_3_qc/1 -> Scope6/1, [Pos_Motor_3_qc]
  Pos_Motor_2_qc/1 -> Scope5/1, [Pos_Motor_2_qc]
  Pos_Motor_1_qc/1 -> Scope/1, [Pos_Motor_1_qc]
  Pos_IncreaseDecrease/1 -> [Pos_IncreaseDecrease]
  [LeftMotor4_RightMotor1] -> Chart2/1(LeftMotor4_RightMotor1)
  [UpMotor3_DownMotor2] -> Chart2/2(UpMotor3_DownMotor2)
  Chart2/1(flag_direction) -> [flag_direction]  "flag_direction"
  Compare To Constant7/1 -> Displacement_mode_flag=0/Enable
  [flag_direction] -> Detect Change2/1
  [flag_direction] -> Displacement_mode_flag=0/6(flag)
  [Pos_Motor_2_qc] -> Displacement_mode_flag=0/2(Pos_Motor_2_qc)
  [Pos_Motor_4_qc] -> Displacement_mode_flag=0/4(Pos_Motor_4_qc)
  [Pos_Motor_1_qc] -> Displacement_mode_flag=0/1(Pos_Motor_1_qc)
  [Pos_Motor_3_qc] -> Displacement_mode_flag=0/3(Pos_Motor_3_qc)
  [flag_direction] -> Compare To Constant7/1
  Detect Change2/1 -> Displacement_mode_flag=0/5(flag_change)
  Displacement_mode_flag=0/1(Motor1PosReq_qc) -> [Motor1PosReq_qc_mode0]
  Displacement_mode_flag=0/2(Motor2_pos_req_qc) -> [Motor2PosReq_qc_mode0]
  Displacement_mode_flag=0/3(Motor3PosReq_qc) -> [Motor3PosReq_qc_mode0]
  Displacement_mode_flag=0/4(Motor4PosReq_qc) -> [Motor4PosReq_qc_mode0]
  Detect Change1/1 -> Displacement_mode_flag=1/6(flag_change)
  [flag_direction] -> Compare To Constant1/1
  [flag_direction] -> Displacement_mode_flag=1/7(flag)
  [flag_direction] -> Detect Change1/1
  Displacement_mode_flag=1/1(Motor1PosReq_qc) -> [Motor1PosReq_qc_mode1]
  [Pos_Motor_3_qc] -> Displacement_mode_flag=1/4(Pos_Motor_3_qc)
  Displacement_mode_flag=1/4(Motor4PosReq_qc) -> [Motor4PosReq_qc_mode1]
  [Pos_Motor_2_qc] -> Displacement_mode_flag=1/3(Pos_Motor_2_qc)
  Displacement_mode_flag=1/3(Motor3PosReq_qc) -> [Motor3PosReq_qc_mode1]
  [Pos_Motor_4_qc] -> Displacement_mode_flag=1/5(Pos_Motor_4_qc)
  Displacement_mode_flag=1/2(Motor2_pos_req_qc) -> [Motor2PosReq_qc_mode1]
  Compare To Constant1/1 -> Displacement_mode_flag=1/Enable
  [Pos_IncreaseDecrease] -> Displacement_mode_flag=1/1(Pos_IncreaseDecrease)
  [Pos_Motor_1_qc] -> Displacement_mode_flag=1/2(Pos_Motor_1_qc)
  Demux2/2 -> Scope1/1, [Motor2PosReq_qc]
  [Motor4PosReq_qc_mode2] -> Mux7/4
  [Motor1PosReq_qc_mode2] -> Mux7/1
  Demux2/3 -> Scope3/1, [Motor3PosReq_qc]
  [Motor2PosReq_qc_mode2] -> Mux7/2
  [flag_direction] -> Multiport Switch1/1
  Multiport Switch1/1 -> Demux2/1
  [Motor1PosReq_qc_mode1] -> Mux6/1
  [Motor4PosReq_qc_mode4] -> Mux10/4
  [Motor3PosReq_qc_mode1] -> Mux6/3
  [Motor3PosReq_qc_mode2] -> Mux7/3
  Demux2/4 -> Scope4/1, [Motor4PosReq_qc]
  [Motor3PosReq_qc_mode4] -> Mux10/3
  [Motor2PosReq_qc_mode1] -> Mux6/2
  [Motor3PosReq_qc_mode3] -> Mux9/3
  [Motor4PosReq_qc_mode3] -> Mux9/4
  [Motor4PosReq_qc_mode1] -> Mux6/4
  [Motor2PosReq_qc_mode3] -> Mux9/2
  [Motor2PosReq_qc_mode4] -> Mux10/2
  [Motor1PosReq_qc_mode4] -> Mux10/1
  [Motor1PosReq_qc_mode3] -> Mux9/1
  Demux2/1 -> Scope2/1, [Motor1PosReq_qc]
  [Pos_Motor_2_qc] -> Displacement_mode_flag=2/3(Pos_Motor_2_qc)
  Compare To Constant2/1 -> Displacement_mode_flag=2/Enable
  Displacement_mode_flag=2/2(Motor2_pos_req_qc) -> [Motor2PosReq_qc_mode2]
  [Pos_Motor_4_qc] -> Displacement_mode_flag=2/5(Pos_Motor_4_qc)
  Displacement_mode_flag=2/4(Motor4PosReq_qc) -> [Motor4PosReq_qc_mode2]
  [Pos_IncreaseDecrease] -> Displacement_mode_flag=2/1(Pos_IncreaseDecrease)
  Displacement_mode_flag=2/3(Motor3PosReq_qc) -> [Motor3PosReq_qc_mode2]
  [flag_direction] -> Compare To Constant2/1
  Displacement_mode_flag=2/1(Motor1PosReq_qc) -> [Motor1PosReq_qc_mode2]
  [Pos_Motor_1_qc] -> Displacement_mode_flag=2/2(Pos_Motor_1_qc)
  [flag_direction] -> Displacement_mode_flag=2/7(flag)
  [flag_direction] -> Detect Change3/1
  [Pos_Motor_3_qc] -> Displacement_mode_flag=2/4(Pos_Motor_3_qc)
  Detect Change3/1 -> Displacement_mode_flag=2/6(flag_change)
  [Pos_Motor_4_qc] -> Displacement_mode_flag=3/5(Pos_Motor_4_qc)
  Displacement_mode_flag=3/2(Motor2_pos_req_qc) -> [Motor2PosReq_qc_mode3]
  Compare To Constant3/1 -> Displacement_mode_flag=3/Enable
  [Pos_Motor_2_qc] -> Displacement_mode_flag=3/3(Pos_Motor_2_qc)
  Displacement_mode_flag=3/4(Motor4PosReq_qc) -> [Motor4PosReq_qc_mode3]
  [Pos_IncreaseDecrease] -> Displacement_mode_flag=3/1(Pos_IncreaseDecrease)
  Detect Change4/1 -> Displacement_mode_flag=3/6(flag_change)
  [flag_direction] -> Displacement_mode_flag=3/7(flag)
  Displacement_mode_flag=3/1(Motor1PosReq_qc) -> [Motor1PosReq_qc_mode3]
  [Pos_Motor_1_qc] -> Displacement_mode_flag=3/2(Pos_Motor_1_qc)
  [flag_direction] -> Compare To Constant3/1
  Displacement_mode_flag=3/3(Motor3PosReq_qc) -> [Motor3PosReq_qc_mode3]
  [Pos_Motor_3_qc] -> Displacement_mode_flag=3/4(Pos_Motor_3_qc)
  [flag_direction] -> Detect Change4/1
  [flag_direction] -> Detect Change5/1
  [Pos_Motor_3_qc] -> Displacement_mode_flag=4/4(Pos_Motor_3_qc)
  Displacement_mode_flag=4/3(Motor3PosReq_qc) -> [Motor3PosReq_qc_mode4]
  [flag_direction] -> Compare To Constant4/1
  [Pos_Motor_1_qc] -> Displacement_mode_flag=4/2(Pos_Motor_1_qc)
  Displacement_mode_flag=4/1(Motor1PosReq_qc) -> [Motor1PosReq_qc_mode4]
  [flag_direction] -> Displacement_mode_flag=4/7(flag)
  Detect Change5/1 -> Displacement_mode_flag=4/6(flag_change)
  [Pos_IncreaseDecrease] -> Displacement_mode_flag=4/1(Pos_IncreaseDecrease)
  Displacement_mode_flag=4/4(Motor4PosReq_qc) -> [Motor4PosReq_qc_mode4]
  [Pos_Motor_2_qc] -> Displacement_mode_flag=4/3(Pos_Motor_2_qc)
  Compare To Constant4/1 -> Displacement_mode_flag=4/Enable
  Displacement_mode_flag=4/2(Motor2_pos_req_qc) -> [Motor2PosReq_qc_mode4]
  [Pos_Motor_4_qc] -> Displacement_mode_flag=4/5(Pos_Motor_4_qc)
  [Motor4PosReq_qc_mode0] -> Mux1/4
  [Motor2PosReq_qc_mode0] -> Mux1/2
  [Motor3PosReq_qc_mode0] -> Mux1/3
  [Motor1PosReq_qc_mode0] -> Mux1/1
  Mux1/1 -> Multiport Switch1/2
  Mux6/1 -> Multiport Switch1/3
  Mux7/1 -> Multiport Switch1/4
  Mux9/1 -> Multiport Switch1/5
  Mux10/1 -> Multiport Switch1/6
  [Motor1PosReq_qc] -> Motor1PosReq_qc/1
  [Motor2PosReq_qc] -> Motor2_pos_req_qc/1
  [Motor3PosReq_qc] -> Motor3PosReq_qc/1
  [Motor4PosReq_qc] -> Motor4PosReq_qc/1
  [reset] -> Detect Change7/1
  Enable/1 -> [reset]
  Detect Change7/1 -> Scope8/1, Chart2/3(reset)  "enable"
